simulink model "multiple_step"  (R2022b)
settings: Solver=VariableStepAuto  StartTime=0.0  StopTime=90  RelTol=1e-3
libraries: fuzblock x2, simulink x1
settings Model: Creator=sophy  LastModifiedBy=sophy

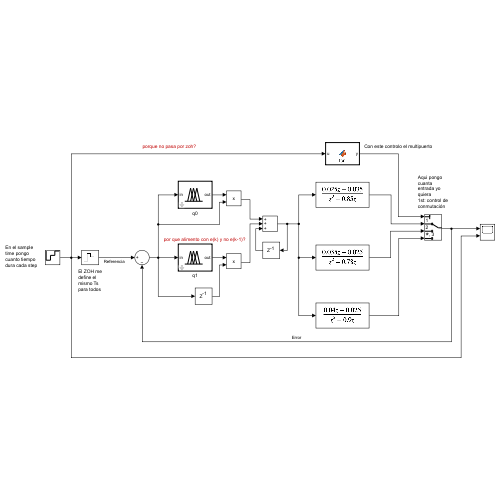
[thumbnail: Simulink's stored preview of the top-level diagram]
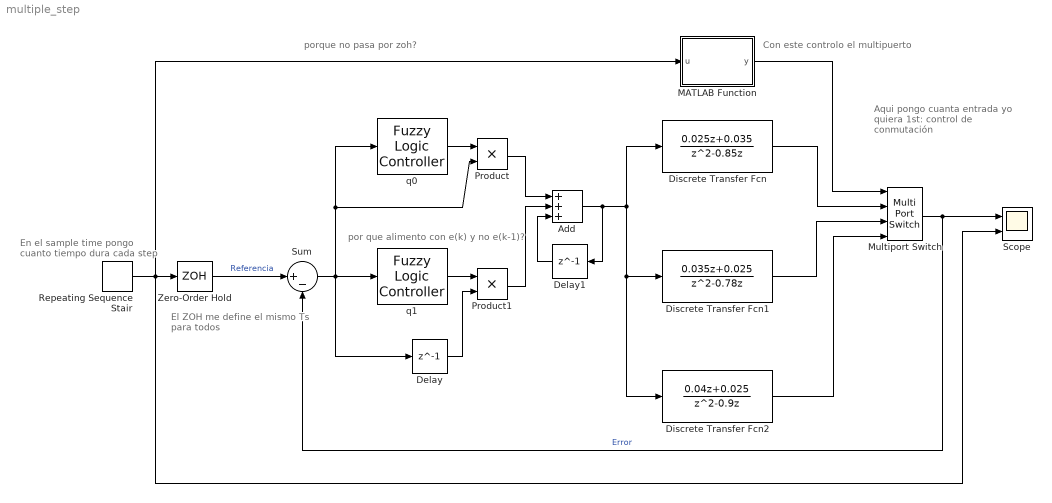
== system multiple_step ==
  note: por que alimento con e(k) y no e(k-1)?
  note: Con este controlo el multipuerto
  note: porque no pasa por zoh?
  note: Aqui pongo cuanta entrada yo quiera
      | 1st: control de conmutación
  note: El ZOH me define el mismo Ts para todos
  note: En el sample time pongo cuanto tiempo dura cada step
  Add : Sum  Inputs=+++
  Delay : Delay  DelayLength=1
  Delay1 : Delay  DelayLength=1
  Discrete Transfer Fcn : DiscreteTransferFcn  Numerator=[0.025 0.035]  Denominator=[1 -0.85 0]
  Discrete Transfer Fcn1 : DiscreteTransferFcn  Numerator=[0.035 0.025]  Denominator=[1 -0.78 0]
  Discrete Transfer Fcn2 : DiscreteTransferFcn  Numerator=[0.04 0.025]  Denominator=[1 -0.9 0]
  MATLAB Function : MATLAB Function  TreatAsAtomicUnit=on
  Multiport Switch : MultiPortSwitch  SaturateOnIntegerOverflow=off  InputSameDT=off
  Product : Product
  Product1 : Product
  Repeating Sequence Stair : simulink/Sources/Repeating Sequence Stair  OutValues=[10 20 30].'  tsamp=30  OutMin=[]  OutMax=[]  OutDataTypeStr=double  OutputDataTypeScalingMode=double  OutDataType=fixdt(0,8)  ConRadixGroup=Best Precision: Vector-wise  OutScaling=2^-12
  Scope : Scope  NumInputPorts=2
  Sum : Sum  Inputs=|+-
  Zero-Order Hold : ZeroOrderHold
  q0 : fuzblock/Fuzzy Logic  Controller  FIS='tipper.fis'  OutputSampleNumber=101  DataType=double  FuzzifiedInputs=off  RuleFiringStrengths=off  RuleOutputs=off  AggregatedOutputs=off  SimulateUsing=Interpreted execution  OutOfRangeInputValueMessage=warning  NoRuleFiredMessage=warning  EmptyOutputFuzzySetMessage=warning
  q1 : fuzblock/Fuzzy Logic  Controller  FIS='tipper.fis'  OutputSampleNumber=101  DataType=double  FuzzifiedInputs=off  RuleFiringStrengths=off  RuleOutputs=off  AggregatedOutputs=off  SimulateUsing=Interpreted execution  OutOfRangeInputValueMessage=warning  NoRuleFiredMessage=warning  EmptyOutputFuzzySetMessage=warning
  wires:
  Repeating Sequence Stair/1 -> Zero-Order Hold/1, Scope/2, MATLAB Function/1(u)
  Zero-Order Hold/1 -> Sum/1  "Referencia"
  MATLAB Function/1(y) -> Multiport Switch/1
  Discrete Transfer Fcn/1 -> Multiport Switch/2
  Discrete Transfer Fcn1/1 -> Multiport Switch/3
  Discrete Transfer Fcn2/1 -> Multiport Switch/4
  Multiport Switch/1 -> Scope/1, Sum/2  "Error"
  Sum/1 -> Delay/1, q1/1, q0/1, Product/2
  q0/1 -> Product/1
  q1/1 -> Product1/1
  Delay/1 -> Product1/2
  Product/1 -> Add/1
  Product1/1 -> Add/2
  Add/1 -> Discrete Transfer Fcn2/1, Discrete Transfer Fcn1/1, Discrete Transfer Fcn/1, Delay1/1
  Delay1/1 -> Add/3

== matlab function multiple_step/MATLAB Function ==
  data: u input; y output
function y = fcn(u)

if ((u>0)&&(u<=10)) % u = lo que entra = escalon
u = 1; % activar pin 1
end

if ((u>10)&&(u<=20))
u = 2; % activar pin 2
end 

if ((u>20)&&(u<=30))
u = 3; % activar pin 3
end 

y = u;
